simulink model "iftest"  (Simulink 7.6)
settings: Solver=ode3  StartTime=0.0  StopTime=10.0  FixedStep=1  RelTol=1e-3
PreLoadFcn:
  | tripleBusObject
settings Model: Creator=hnine  LastModifiedBy=c2wt
settings DataIOCC: SignalLogging=off
settings OptimizationCC: InitFltsAndDblsToZero=on
settings DebuggingCC: SaveWithParameterizedLinksMsg=none  BusObjectLabelMismatch=none  StrictBusMsg=Warning
settings GRTTargetCC: TargetFcnLib=ansi_tfl_tmw.mat

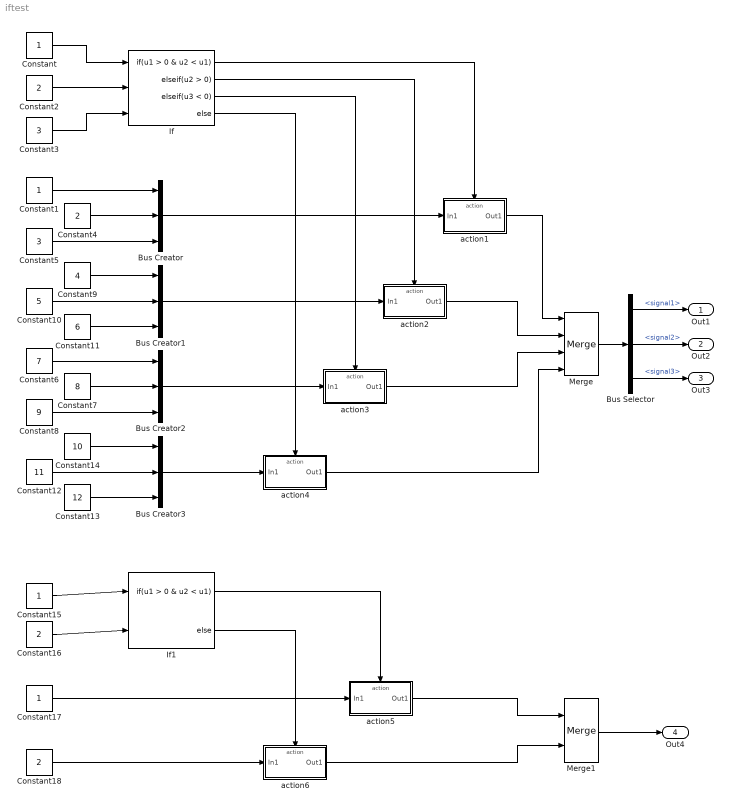
== system iftest ==
  Bus Creator{,1..3} (4 alike) : BusCreator  Inputs=3  OutDataTypeStr=Bus: triple  NonVirtualBus=on
  Bus Selector : BusSelector  OutputSignals=signal1,signal2,signal3
  Constant{,1,15,17} (4 alike) : Constant
  Constant10 : Constant  Value=5
  Constant11 : Constant  Value=6
  Constant12 : Constant  Value=11
  Constant13 : Constant  Value=12
  Constant14 : Constant  Value=10
  Constant{2,4,16,18} (4 alike) : Constant  Value=2
  Constant3 : Constant  Value=3
  Constant5 : Constant  Value=3
  Constant6 : Constant  Value=7
  Constant7 : Constant  Value=8
  Constant8 : Constant  Value=9
  Constant9 : Constant  Value=4
  If : If  NumInputs=3  IfExpression=u1 > 0 & u2 < u1  ElseIfExpressions=u2 > 0, u3 < 0  ZeroCross=off
  If1 : If  NumInputs=2  IfExpression=u1 > 0 & u2 < u1  ZeroCross=off
  Merge : Merge  Inputs=4  InputPortOffsets=[ 0 3 6 9 ]
  Merge1 : Merge  InputPortOffsets=[ 0 3 6 9 ]
  action1 : Subsystem  TreatAsAtomicUnit=on
  action2 : Subsystem  TreatAsAtomicUnit=on
  action3 : Subsystem  TreatAsAtomicUnit=on
  action4 : Subsystem  TreatAsAtomicUnit=on
  action5 : Subsystem  TreatAsAtomicUnit=on
  action6 : Subsystem  TreatAsAtomicUnit=on
  Out1 : Outport
  Out2 : Outport  Port=2
  Out3 : Outport  Port=3
  Out4 : Outport  Port=4
  wires:
  Constant/1 -> If/1
  Constant2/1 -> If/2
  Constant3/1 -> If/3
  If/1 -> action1/Action
  If/2 -> action2/Action
  If/3 -> action3/Action
  If/4 -> action4/Action
  action1/1(Out1) -> Merge/1
  action2/1(Out1) -> Merge/2
  action3/1(Out1) -> Merge/3
  action4/1(Out1) -> Merge/4
  Constant1/1 -> Bus Creator/1
  Constant4/1 -> Bus Creator/2
  Constant5/1 -> Bus Creator/3
  Bus Creator/1 -> action1/1(In1)
  Constant6/1 -> Bus Creator2/1
  Constant7/1 -> Bus Creator2/2
  Constant8/1 -> Bus Creator2/3
  Constant9/1 -> Bus Creator1/1
  Constant10/1 -> Bus Creator1/2
  Constant11/1 -> Bus Creator1/3
  Constant14/1 -> Bus Creator3/1
  Constant12/1 -> Bus Creator3/2
  Constant13/1 -> Bus Creator3/3
  Bus Creator1/1 -> action2/1(In1)
  Bus Creator2/1 -> action3/1(In1)
  Bus Creator3/1 -> action4/1(In1)
  Merge/1 -> Bus Selector/1
  Bus Selector/1 -> Out1/1  "<signal1>"
  Bus Selector/2 -> Out2/1  "<signal2>"
  Bus Selector/3 -> Out3/1  "<signal3>"
  Constant15/1 -> If1/1
  Constant16/1 -> If1/2
  Constant17/1 -> action5/1(In1)
  Constant18/1 -> action6/1(In1)
  If1/1 -> action5/Action
  If1/2 -> action6/Action
  action5/1(Out1) -> Merge1/1
  action6/1(Out1) -> Merge1/2
  Merge1/1 -> Out4/1

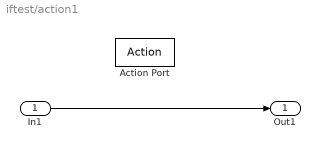
== system iftest/action1 ==
  In1 : Inport
  Action Port : ActionPort  ActionType=then
  Out1 : Outport
  wires:
  In1/1 -> Out1/1

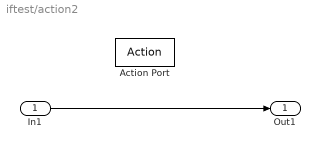
== system iftest/action2 ==
  In1 : Inport
  Action Port : ActionPort  ActionType=elseif
  Out1 : Outport
  wires:
  In1/1 -> Out1/1

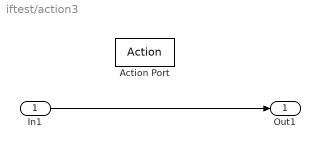
== system iftest/action3 ==
  In1 : Inport
  Action Port : ActionPort  ActionType=elseif
  Out1 : Outport
  wires:
  In1/1 -> Out1/1

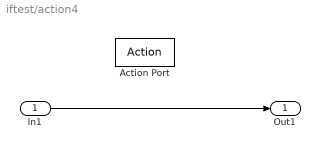
== system iftest/action4 ==
  In1 : Inport
  Action Port : ActionPort  ActionType=else
  Out1 : Outport
  wires:
  In1/1 -> Out1/1

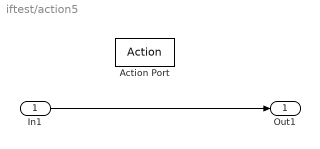
== system iftest/action5 ==
  In1 : Inport
  Action Port : ActionPort  ActionType=then
  Out1 : Outport
  wires:
  In1/1 -> Out1/1

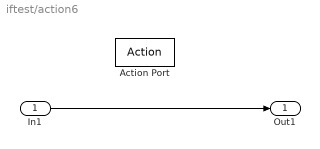
== system iftest/action6 ==
  In1 : Inport
  Action Port : ActionPort  ActionType=else
  Out1 : Outport
  wires:
  In1/1 -> Out1/1
